simulink model "injection_timing_model"  (R2026a)
settings: Solver=VariableStepAuto  StopTime=300
undefined symbols (not defined in the file): engine
settings Model: Creator=GOD  LastModifiedBy=GOD

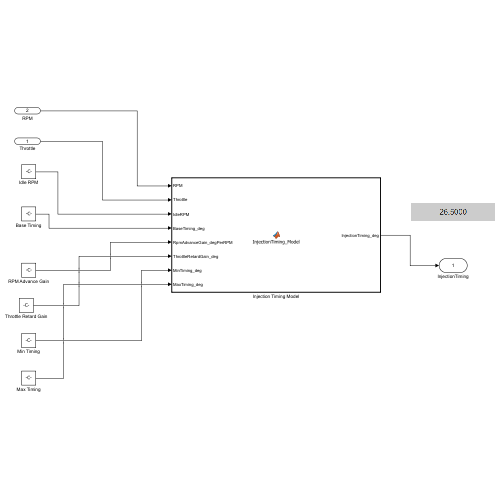
[thumbnail: Simulink's stored preview of the top-level diagram]
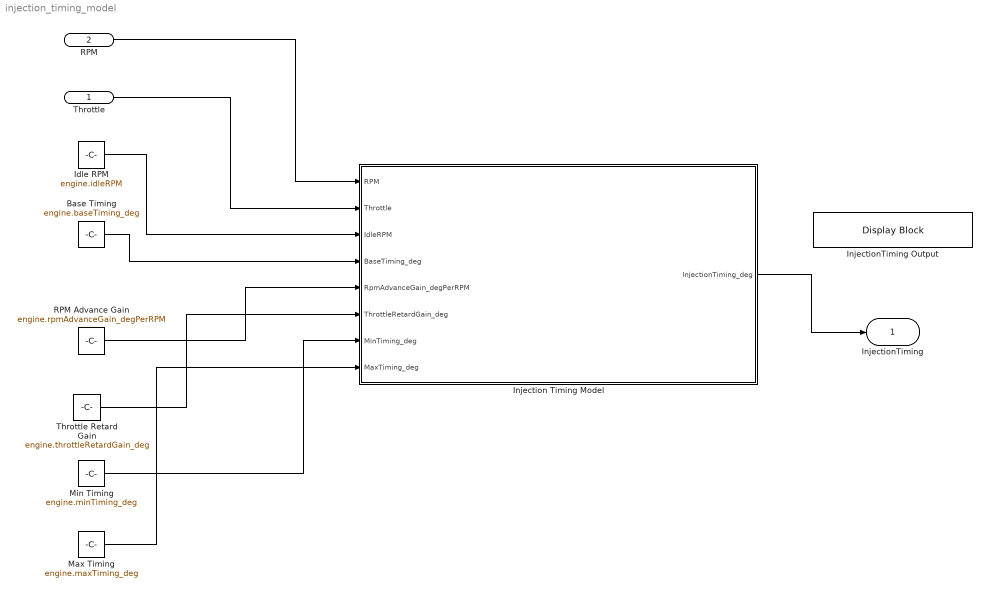
== system injection_timing_model ==
  Throttle : Inport
  RPM : Inport  Port=2
  Base Timing : Constant  Value=engine.baseTiming_deg
  Idle RPM : Constant  Value=engine.idleRPM
  Injection Timing Model : MATLAB Function  TreatAsAtomicUnit=on
  InjectionTiming Output : DisplayBlock  LabelPosition=Hide  Transparency=1  GridColor=[0.502, 0.502, 0.502]
  Max Timing : Constant  Value=engine.maxTiming_deg
  Min Timing : Constant  Value=engine.minTiming_deg
  RPM Advance Gain : Constant  Value=engine.rpmAdvanceGain_degPerRPM
  Throttle Retard Gain : Constant  Value=engine.throttleRetardGain_deg
  InjectionTiming : Outport
  wires:
  Idle RPM/1 -> Injection Timing Model/3(IdleRPM)
  Base Timing/1 -> Injection Timing Model/4(BaseTiming_deg)
  RPM Advance Gain/1 -> Injection Timing Model/5(RpmAdvanceGain_degPerRPM)
  Throttle Retard Gain/1 -> Injection Timing Model/6(ThrottleRetardGain_deg)
  Min Timing/1 -> Injection Timing Model/7(MinTiming_deg)
  Max Timing/1 -> Injection Timing Model/8(MaxTiming_deg)
  Injection Timing Model/1(InjectionTiming_deg) -> InjectionTiming/1
  RPM/1 -> Injection Timing Model/1(RPM)
  Throttle/1 -> Injection Timing Model/2(Throttle)

== matlab function injection_timing_model/Injection Timing Model ==
  data: RPM input; InjectionTiming_deg output; Throttle input; IdleRPM input; BaseTiming_deg input; RpmAdvanceGain_degPerRPM input; ThrottleRetardGain_deg input; MinTiming_deg input; MaxTiming_deg input
function InjectionTiming_deg = InjectionTiming_Model(RPM, Throttle, ...
                                    IdleRPM, BaseTiming_deg, RpmAdvanceGain_degPerRPM, ...
                                    ThrottleRetardGain_deg, MinTiming_deg, MaxTiming_deg)
% Engineering-assumption injection/ignition timing model.
% Timing advances with RPM above idle, and retards slightly under
% heavy throttle (a simple stand-in for knock/enrichment protection).
timing = BaseTiming_deg + RpmAdvanceGain_degPerRPM * (RPM - IdleRPM) ...
    - ThrottleRetardGain_deg * Throttle;
if timing < MinTiming_deg
    timing = MinTiming_deg;
elseif timing > MaxTiming_deg
    timing = MaxTiming_deg;
end
InjectionTiming_deg = timing;
end
